simulink model "ddsfloat"  (R2018b)
settings: Solver=VariableStepAuto  StartTime=0.0  StopTime=10000E-6  RelTol=1e-3
settings Model: Creator=caeuser  LastModifiedBy=caeuser

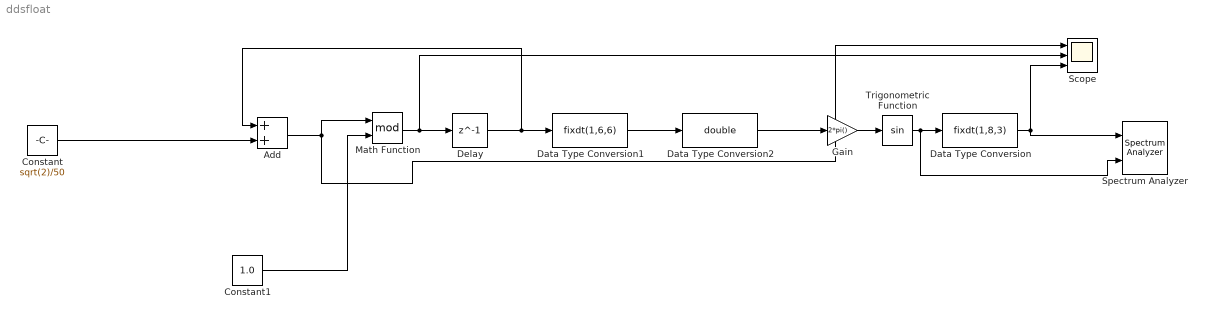
== system ddsfloat ==
  Add : Sum
  Constant : Constant  Value=sqrt(2)/50  SampleTime=20E-9
  Constant1 : Constant  Value=1.0  SampleTime=20E-9
  Data Type Conversion : DataTypeConversion  OutDataTypeStr=fixdt(1,8,3)
  Data Type Conversion1 : DataTypeConversion  OutDataTypeStr=fixdt(1,6,6)
  Data Type Conversion2 : DataTypeConversion  OutDataTypeStr=double
  Delay : Delay  DelayLength=1
  Gain : Gain  Gain=2*pi()
  Math Function : Math  Operator=mod  SaturateOnIntegerOverflow=on
  Scope : Scope  NumInputPorts=3
  Spectrum Analyzer : SpectrumAnalyzer  NumInputPorts=2
  Trigonometric Function : Trigonometry
  wires:
  Gain/1 -> Trigonometric Function/1
  Add/1 -> Scope/1, Math Function/1
  Math Function/1 -> Scope/2, Delay/1
  Delay/1 -> Data Type Conversion1/1, Add/1
  Trigonometric Function/1 -> Spectrum Analyzer/2, Data Type Conversion/1
  Constant1/1 -> Math Function/2
  Constant/1 -> Add/2
  Data Type Conversion/1 -> Scope/3, Spectrum Analyzer/1
  Data Type Conversion1/1 -> Data Type Conversion2/1
  Data Type Conversion2/1 -> Gain/1
